simulink library "sumTetherForcesAndMoments"  (R2018b)
settings: Solver=VariableStepAuto  StartTime=0.0  StopTime=10.0  RelTol=1e-3
values from neighbouring files (symbols this model uses):
  attchPtMat = zeros(3,numTethers)    [sumTetherForcesAndMoments_init.m]
  numTethers = length(thr_struct)    [sumTetherForcesAndMoments_init.m]
undefined symbols (not defined in the file or in its folder): class_thr
libraries: vrlib x1, eulAng2RotMat_ul x1
settings Model: Creator=Ayaz  LastModifiedBy=Ayaz

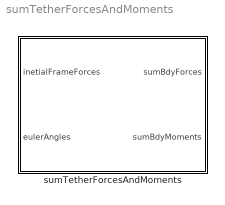
== system sumTetherForcesAndMoments ==
  sumTetherForcesAndMoments : Subsystem  TreatAsAtomicUnit=on  mask{thr_struct=class_thr, attach_point=ground station}
      mask prompts: thr_struct "Tether field"; attach_point "Choose attachment point"
      mask init:
      | % initialization script
      | sumTetherForcesAndMoments_init
      mask TypeOptions attach_point: ground station | lifting body

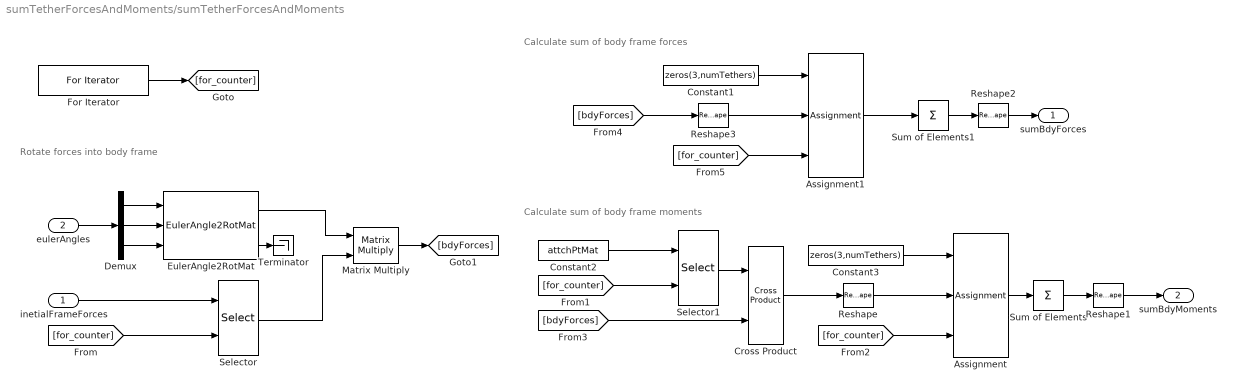
== system sumTetherForcesAndMoments/sumTetherForcesAndMoments ==
  note: Calculate sum of body frame forces
  note: Rotate forces into body frame
  note: Calculate sum of body frame moments
  inetialFrameForces : Inport
  eulerAngles : Inport  Port=2
  Assignment : Assignment  NumberOfDimensions=2  DiagnosticForDimensions=Warning  IndexOptions=Assign all,Index vector (port)  Indices=1,1  OutputSizes=1,1
  Assignment1 : Assignment  NumberOfDimensions=2  DiagnosticForDimensions=Warning  IndexOptions=Assign all,Index vector (port)  Indices=1,1  OutputSizes=1,1
  Constant1 : Constant  Value=zeros(3,numTethers)
  Constant2 : Constant  Value=attchPtMat
  Constant3 : Constant  Value=zeros(3,numTethers)
  Cross Product : vrlib/Utilities/Cross Product
      settings: SourceProductBaseCode=VR
  Demux : Demux  Outputs=3
  EulerAngle2RotMat : eulAng2RotMat_ul/EulerAngle2RotMat  SystemSampleTime=-1
  For Iterator : ForIterator  IterationLimit=numTethers
  Matrix Multiply : Product  Multiplication=Matrix(*)
  Reshape{,1..3} (4 alike) : Reshape  OutputDimensionality=Column vector (2-D)
  Selector : Selector  NumberOfDimensions=2  InputPortWidth=3  IndexOptions=Select all,Index vector (port)  Indices=[1 3],1  OutputSizes=1,1
  Selector1 : Selector  NumberOfDimensions=2  InputPortWidth=3  IndexOptions=Select all,Index vector (port)  Indices=[1 3],1  OutputSizes=1,1
  Sum of Elements : Sum  Inputs=+  CollapseMode=Specified dimension  CollapseDim=2
  Sum of Elements1 : Sum  Inputs=+  CollapseMode=Specified dimension  CollapseDim=2
  Terminator : Terminator
  sumBdyForces : Outport
  sumBdyMoments : Outport  Port=2
  wires:
  eulerAngles/1 -> Demux/1
  Demux/2 -> EulerAngle2RotMat/2
  Demux/1 -> EulerAngle2RotMat/1
  EulerAngle2RotMat/2 -> Terminator/1
  Reshape1/1 -> sumBdyMoments/1
  Matrix Multiply/1 -> [bdyForces]
  [for_counter] -> Selector1/2
  Constant3/1 -> Assignment/1
  Demux/3 -> EulerAngle2RotMat/3
  [for_counter] -> Assignment/3
  Selector1/1 -> Cross Product/1
  Cross Product/1 -> Reshape/1
  Reshape/1 -> Assignment/2
  EulerAngle2RotMat/1 -> Matrix Multiply/1
  Sum of Elements1/1 -> Reshape2/1
  Constant2/1 -> Selector1/1
  Reshape2/1 -> sumBdyForces/1
  Selector/1 -> Matrix Multiply/2
  [for_counter] -> Selector/2
  Assignment/1 -> Sum of Elements/1
  Sum of Elements/1 -> Reshape1/1
  inetialFrameForces/1 -> Selector/1
  [bdyForces] -> Cross Product/2
  For Iterator/1 -> [for_counter]
  Reshape3/1 -> Assignment1/2
  [for_counter] -> Assignment1/3
  [bdyForces] -> Reshape3/1
  Constant1/1 -> Assignment1/1
  Assignment1/1 -> Sum of Elements1/1
